simulink model "Sim7"  (R2019a)
settings: Solver=VariableStepAuto  StartTime=0.0  StopTime=10.0  RelTol=1e-2
settings Model: Creator=fbleo  LastModifiedBy=fbleo

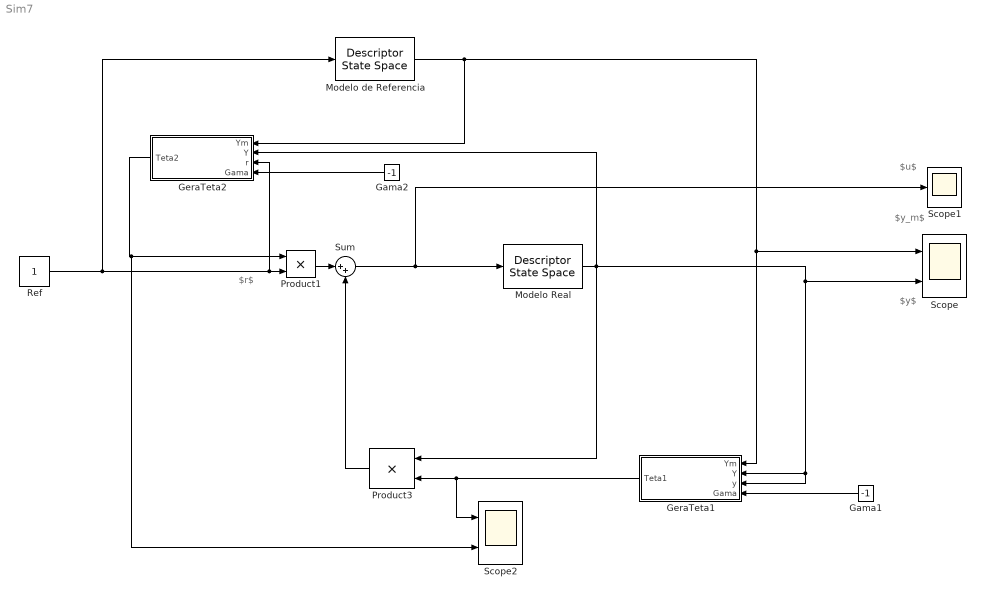
== system Sim7 ==
  note: $y$
  note: $y_m$
  note: $u$
  note: $r$
  Gama1 : Constant  Value=-1
  Gama2 : Constant  Value=-1
  GeraTeta1 : Subsystem
  GeraTeta2 : Subsystem
  Modelo Real : DescriptorStateSpace  A=-1  B=2  D=0  InitialCondition=0.5
  Modelo de Referencia : DescriptorStateSpace  A=-3  B=3  D=0  InitialCondition=0
  Product1 : Product
  Product3 : Product
  Ref : Constant
  Scope : Scope  NumInputPorts=2
  Scope1 : Scope
  Scope2 : Scope  NumInputPorts=2
  Sum : Sum  Inputs=|++
  wires:
  Product3/1 -> Sum/2
  Sum/1 -> Scope1/1, Modelo Real/1
  Ref/1 -> GeraTeta2/3(r), Product1/2, Modelo de Referencia/1
  Modelo Real/1 -> Scope/2, GeraTeta1/3(y), GeraTeta1/2(Y), Product3/1, GeraTeta2/2(Y)
  Product1/1 -> Sum/1
  Modelo de Referencia/1 -> GeraTeta1/1(Ym), Scope/1, GeraTeta2/1(Ym)
  Gama1/1 -> GeraTeta1/4(Gama)
  GeraTeta1/1(Teta1) -> Scope2/1, Product3/2
  Gama2/1 -> GeraTeta2/4(Gama)
  GeraTeta2/1(Teta2) -> Scope2/2, Product1/1

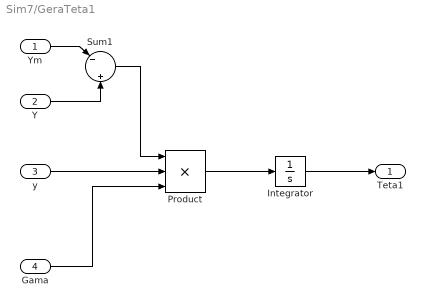
== system Sim7/GeraTeta1 ==
  Ym : Inport
  Y : Inport  Port=2
  y : Inport  Port=3
  Gama : Inport  Port=4
  Integrator : Integrator  InitialCondition=-0.65
  Product : Product  Inputs=3
  Sum1 : Sum  Inputs=|-||+
  Teta1 : Outport
  wires:
  Ym/1 -> Sum1/1
  Y/1 -> Sum1/2
  Sum1/1 -> Product/1
  y/1 -> Product/2
  Gama/1 -> Product/3
  Product/1 -> Integrator/1
  Integrator/1 -> Teta1/1

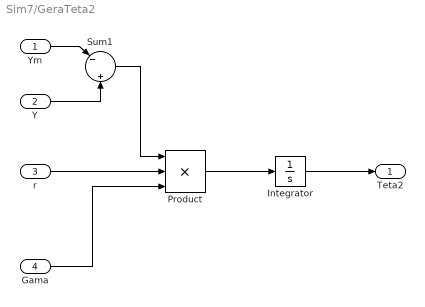
== system Sim7/GeraTeta2 ==
  Ym : Inport
  Y : Inport  Port=2
  r : Inport  Port=3
  Gama : Inport  Port=4
  Integrator : Integrator  InitialCondition=1.14
  Product : Product  Inputs=3
  Sum1 : Sum  Inputs=|-||+
  Teta2 : Outport
  wires:
  Ym/1 -> Sum1/1
  Y/1 -> Sum1/2
  Sum1/1 -> Product/1
  r/1 -> Product/2
  Gama/1 -> Product/3
  Product/1 -> Integrator/1
  Integrator/1 -> Teta2/1
